simulink model "Parallel_n64"  (R2012b)
settings: Solver=VariableStepDiscrete  StartTime=0.0  StopTime=TotalIterations  RelTol=1e-3
values from neighbouring files (symbols this model uses):
  bp = 12    [ConfigValidate.m]
  bpSNMemory = bp    (= 12)    [ConfigValidate.m]
  IterationsOrdering = 4000    [ConfigValidate.m]
  MaxCoordDistance = (abs(max(wx) - min(wx))+abs(max(wy) - min(wy)))^2    [ConfigValidate.m]
  N_limit = 0.01    [ConfigValidate.m]
  nBits = 9    [ConfigValidate.m]
  nBitsNSmemories = (ceil(log2(TotalIterations)))    [ConfigValidate.m]
  S_limit = 1    [ConfigValidate.m]
  SourceNodes = 2000    [ConfigValidate.m]
  ts = 1    [ConfigValidate.m]
  w1 = rand(1,Neurons)    [ConfigValidate.m]
  w2 = rand(1,Neurons)    [ConfigValidate.m]
  wx = zeros(1,Neurons)    [ConfigValidate.m]
  wy = zeros(1,Neurons)    [ConfigValidate.m]
  x1 = rand(SourceNodes,1)    [ConfigValidate.m]
  x2 = rand(SourceNodes,1)    [ConfigValidate.m]
libraries: xbsIndex_r4 x6367, dspsrcs4 x2, dspstat3 x2
(part 2 of 28)

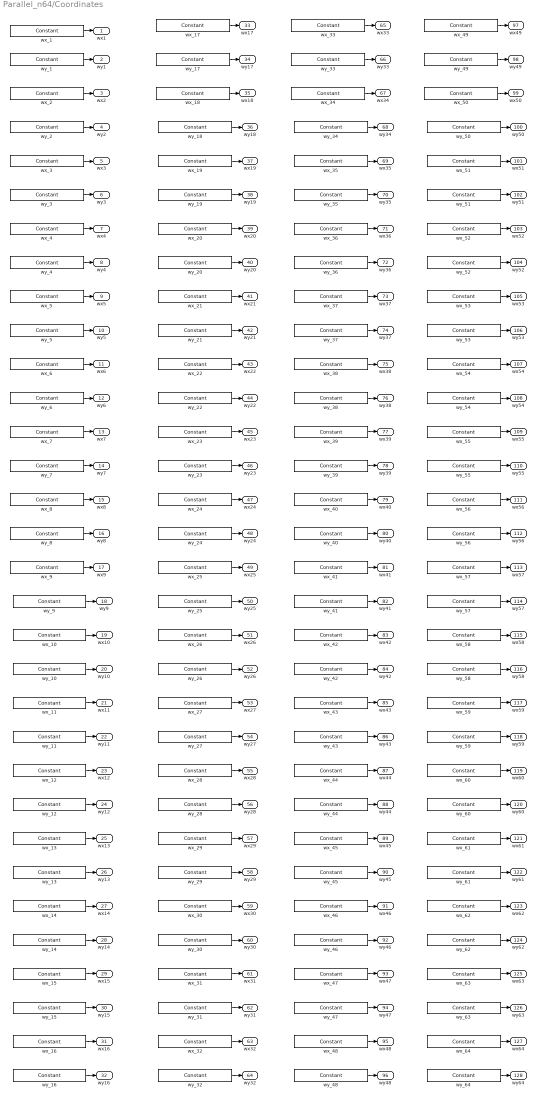
== system Parallel_n64/Coordinates ==
  wx_1 : xbsIndex_r4/Constant  const=wx(1)  gui_display_data_type=Fixed-point  arith_type=Unsigned  n_bits=nbCoord  bin_pt=bpCoord  preci_type=Single  exp_width=8  frac_width=24  explicit_period=on  period=ts  equ=P=C  opselect=C  inp2=PCIN>>17  opr=+  inp1=P  carry=CIN  dbl_ovrd=off  block_type=constant
  wx_{10,26,42,58} (4 alike) : xbsIndex_r4/Constant  const=wx(10)  gui_display_data_type=Fixed-point  arith_type=Unsigned  n_bits=nbCoord  bin_pt=bpCoord  preci_type=Single  exp_width=8  frac_width=24  explicit_period=on  period=ts  equ=P=C  opselect=C  inp2=PCIN>>17  opr=+  inp1=P  carry=CIN  dbl_ovrd=off  block_type=constant
  wx_{11,27,43,59} (4 alike) : xbsIndex_r4/Constant  const=wx(11)  gui_display_data_type=Fixed-point  arith_type=Unsigned  n_bits=nbCoord  bin_pt=bpCoord  preci_type=Single  exp_width=8  frac_width=24  explicit_period=on  period=ts  equ=P=C  opselect=C  inp2=PCIN>>17  opr=+  inp1=P  carry=CIN  dbl_ovrd=off  block_type=constant
  wx_{12,28,44,60} (4 alike) : xbsIndex_r4/Constant  const=wx(12)  gui_display_data_type=Fixed-point  arith_type=Unsigned  n_bits=nbCoord  bin_pt=bpCoord  preci_type=Single  exp_width=8  frac_width=24  explicit_period=on  period=ts  equ=P=C  opselect=C  inp2=PCIN>>17  opr=+  inp1=P  carry=CIN  dbl_ovrd=off  block_type=constant
  wx_{13,29,45,61} (4 alike) : xbsIndex_r4/Constant  const=wx(13)  gui_display_data_type=Fixed-point  arith_type=Unsigned  n_bits=nbCoord  bin_pt=bpCoord  preci_type=Single  exp_width=8  frac_width=24  explicit_period=on  period=ts  equ=P=C  opselect=C  inp2=PCIN>>17  opr=+  inp1=P  carry=CIN  dbl_ovrd=off  block_type=constant
  wx_{14,30,46,62} (4 alike) : xbsIndex_r4/Constant  const=wx(14)  gui_display_data_type=Fixed-point  arith_type=Unsigned  n_bits=nbCoord  bin_pt=bpCoord  preci_type=Single  exp_width=8  frac_width=24  explicit_period=on  period=ts  equ=P=C  opselect=C  inp2=PCIN>>17  opr=+  inp1=P  carry=CIN  dbl_ovrd=off  block_type=constant
  wx_{15,31,47,63} (4 alike) : xbsIndex_r4/Constant  const=wx(15)  gui_display_data_type=Fixed-point  arith_type=Unsigned  n_bits=nbCoord  bin_pt=bpCoord  preci_type=Single  exp_width=8  frac_width=24  explicit_period=on  period=ts  equ=P=C  opselect=C  inp2=PCIN>>17  opr=+  inp1=P  carry=CIN  dbl_ovrd=off  block_type=constant
  wx_{16,32,48,64} (4 alike) : xbsIndex_r4/Constant  const=wx(16)  gui_display_data_type=Fixed-point  arith_type=Unsigned  n_bits=nbCoord  bin_pt=bpCoord  preci_type=Single  exp_width=8  frac_width=24  explicit_period=on  period=ts  equ=P=C  opselect=C  inp2=PCIN>>17  opr=+  inp1=P  carry=CIN  dbl_ovrd=off  block_type=constant
  wx_17 : xbsIndex_r4/Constant  const=wx(17)  gui_display_data_type=Fixed-point  arith_type=Unsigned  n_bits=nbCoord  bin_pt=bpCoord  preci_type=Single  exp_width=8  frac_width=24  explicit_period=on  period=ts  equ=P=C  opselect=C  inp2=PCIN>>17  opr=+  inp1=P  carry=CIN  dbl_ovrd=off  block_type=constant
  wx_18 : xbsIndex_r4/Constant  const=wx(18)  gui_display_data_type=Fixed-point  arith_type=Unsigned  n_bits=nbCoord  bin_pt=bpCoord  preci_type=Single  exp_width=8  frac_width=24  explicit_period=on  period=ts  equ=P=C  opselect=C  inp2=PCIN>>17  opr=+  inp1=P  carry=CIN  dbl_ovrd=off  block_type=constant
  wx_19 : xbsIndex_r4/Constant  const=wx(19)  gui_display_data_type=Fixed-point  arith_type=Unsigned  n_bits=nbCoord  bin_pt=bpCoord  preci_type=Single  exp_width=8  frac_width=24  explicit_period=on  period=ts  equ=P=C  opselect=C  inp2=PCIN>>17  opr=+  inp1=P  carry=CIN  dbl_ovrd=off  block_type=constant
  wx_2 : xbsIndex_r4/Constant  const=wx(2)  gui_display_data_type=Fixed-point  arith_type=Unsigned  n_bits=nbCoord  bin_pt=bpCoord  preci_type=Single  exp_width=8  frac_width=24  explicit_period=on  period=ts  equ=P=C  opselect=C  inp2=PCIN>>17  opr=+  inp1=P  carry=CIN  dbl_ovrd=off  block_type=constant
  wx_20 : xbsIndex_r4/Constant  const=wx(20)  gui_display_data_type=Fixed-point  arith_type=Unsigned  n_bits=nbCoord  bin_pt=bpCoord  preci_type=Single  exp_width=8  frac_width=24  explicit_period=on  period=ts  equ=P=C  opselect=C  inp2=PCIN>>17  opr=+  inp1=P  carry=CIN  dbl_ovrd=off  block_type=constant
  wx_21 : xbsIndex_r4/Constant  const=wx(21)  gui_display_data_type=Fixed-point  arith_type=Unsigned  n_bits=nbCoord  bin_pt=bpCoord  preci_type=Single  exp_width=8  frac_width=24  explicit_period=on  period=ts  equ=P=C  opselect=C  inp2=PCIN>>17  opr=+  inp1=P  carry=CIN  dbl_ovrd=off  block_type=constant
  wx_22 : xbsIndex_r4/Constant  const=wx(22)  gui_display_data_type=Fixed-point  arith_type=Unsigned  n_bits=nbCoord  bin_pt=bpCoord  preci_type=Single  exp_width=8  frac_width=24  explicit_period=on  period=ts  equ=P=C  opselect=C  inp2=PCIN>>17  opr=+  inp1=P  carry=CIN  dbl_ovrd=off  block_type=constant
  wx_23 : xbsIndex_r4/Constant  const=wx(23)  gui_display_data_type=Fixed-point  arith_type=Unsigned  n_bits=nbCoord  bin_pt=bpCoord  preci_type=Single  exp_width=8  frac_width=24  explicit_period=on  period=ts  equ=P=C  opselect=C  inp2=PCIN>>17  opr=+  inp1=P  carry=CIN  dbl_ovrd=off  block_type=constant
  wx_24 : xbsIndex_r4/Constant  const=wx(24)  gui_display_data_type=Fixed-point  arith_type=Unsigned  n_bits=nbCoord  bin_pt=bpCoord  preci_type=Single  exp_width=8  frac_width=24  explicit_period=on  period=ts  equ=P=C  opselect=C  inp2=PCIN>>17  opr=+  inp1=P  carry=CIN  dbl_ovrd=off  block_type=constant
  wx_25 : xbsIndex_r4/Constant  const=wx(25)  gui_display_data_type=Fixed-point  arith_type=Unsigned  n_bits=nbCoord  bin_pt=bpCoord  preci_type=Single  exp_width=8  frac_width=24  explicit_period=on  period=ts  equ=P=C  opselect=C  inp2=PCIN>>17  opr=+  inp1=P  carry=CIN  dbl_ovrd=off  block_type=constant
  wx_3 : xbsIndex_r4/Constant  const=wx(3)  gui_display_data_type=Fixed-point  arith_type=Unsigned  n_bits=nbCoord  bin_pt=bpCoord  preci_type=Single  exp_width=8  frac_width=24  explicit_period=on  period=ts  equ=P=C  opselect=C  inp2=PCIN>>17  opr=+  inp1=P  carry=CIN  dbl_ovrd=off  block_type=constant
  wx_33 : xbsIndex_r4/Constant  const=wx(17)  gui_display_data_type=Fixed-point  arith_type=Unsigned  n_bits=nbCoord  bin_pt=bpCoord  preci_type=Single  exp_width=8  frac_width=24  explicit_period=on  period=ts  equ=P=C  opselect=C  inp2=PCIN>>17  opr=+  inp1=P  carry=CIN  dbl_ovrd=off  block_type=constant
  wx_34 : xbsIndex_r4/Constant  const=wx(18)  gui_display_data_type=Fixed-point  arith_type=Unsigned  n_bits=nbCoord  bin_pt=bpCoord  preci_type=Single  exp_width=8  frac_width=24  explicit_period=on  period=ts  equ=P=C  opselect=C  inp2=PCIN>>17  opr=+  inp1=P  carry=CIN  dbl_ovrd=off  block_type=constant
  wx_35 : xbsIndex_r4/Constant  const=wx(19)  gui_display_data_type=Fixed-point  arith_type=Unsigned  n_bits=nbCoord  bin_pt=bpCoord  preci_type=Single  exp_width=8  frac_width=24  explicit_period=on  period=ts  equ=P=C  opselect=C  inp2=PCIN>>17  opr=+  inp1=P  carry=CIN  dbl_ovrd=off  block_type=constant
  wx_36 : xbsIndex_r4/Constant  const=wx(20)  gui_display_data_type=Fixed-point  arith_type=Unsigned  n_bits=nbCoord  bin_pt=bpCoord  preci_type=Single  exp_width=8  frac_width=24  explicit_period=on  period=ts  equ=P=C  opselect=C  inp2=PCIN>>17  opr=+  inp1=P  carry=CIN  dbl_ovrd=off  block_type=constant
  wx_37 : xbsIndex_r4/Constant  const=wx(21)  gui_display_data_type=Fixed-point  arith_type=Unsigned  n_bits=nbCoord  bin_pt=bpCoord  preci_type=Single  exp_width=8  frac_width=24  explicit_period=on  period=ts  equ=P=C  opselect=C  inp2=PCIN>>17  opr=+  inp1=P  carry=CIN  dbl_ovrd=off  block_type=constant
  wx_38 : xbsIndex_r4/Constant  const=wx(22)  gui_display_data_type=Fixed-point  arith_type=Unsigned  n_bits=nbCoord  bin_pt=bpCoord  preci_type=Single  exp_width=8  frac_width=24  explicit_period=on  period=ts  equ=P=C  opselect=C  inp2=PCIN>>17  opr=+  inp1=P  carry=CIN  dbl_ovrd=off  block_type=constant
  wx_39 : xbsIndex_r4/Constant  const=wx(23)  gui_display_data_type=Fixed-point  arith_type=Unsigned  n_bits=nbCoord  bin_pt=bpCoord  preci_type=Single  exp_width=8  frac_width=24  explicit_period=on  period=ts  equ=P=C  opselect=C  inp2=PCIN>>17  opr=+  inp1=P  carry=CIN  dbl_ovrd=off  block_type=constant
  wx_4 : xbsIndex_r4/Constant  const=wx(4)  gui_display_data_type=Fixed-point  arith_type=Unsigned  n_bits=nbCoord  bin_pt=bpCoord  preci_type=Single  exp_width=8  frac_width=24  explicit_period=on  period=ts  equ=P=C  opselect=C  inp2=PCIN>>17  opr=+  inp1=P  carry=CIN  dbl_ovrd=off  block_type=constant
  wx_40 : xbsIndex_r4/Constant  const=wx(24)  gui_display_data_type=Fixed-point  arith_type=Unsigned  n_bits=nbCoord  bin_pt=bpCoord  preci_type=Single  exp_width=8  frac_width=24  explicit_period=on  period=ts  equ=P=C  opselect=C  inp2=PCIN>>17  opr=+  inp1=P  carry=CIN  dbl_ovrd=off  block_type=constant
  wx_41 : xbsIndex_r4/Constant  const=wx(25)  gui_display_data_type=Fixed-point  arith_type=Unsigned  n_bits=nbCoord  bin_pt=bpCoord  preci_type=Single  exp_width=8  frac_width=24  explicit_period=on  period=ts  equ=P=C  opselect=C  inp2=PCIN>>17  opr=+  inp1=P  carry=CIN  dbl_ovrd=off  block_type=constant
  wx_49 : xbsIndex_r4/Constant  const=wx(17)  gui_display_data_type=Fixed-point  arith_type=Unsigned  n_bits=nbCoord  bin_pt=bpCoord  preci_type=Single  exp_width=8  frac_width=24  explicit_period=on  period=ts  equ=P=C  opselect=C  inp2=PCIN>>17  opr=+  inp1=P  carry=CIN  dbl_ovrd=off  block_type=constant
  wx_5 : xbsIndex_r4/Constant  const=wx(5)  gui_display_data_type=Fixed-point  arith_type=Unsigned  n_bits=nbCoord  bin_pt=bpCoord  preci_type=Single  exp_width=8  frac_width=24  explicit_period=on  period=ts  equ=P=C  opselect=C  inp2=PCIN>>17  opr=+  inp1=P  carry=CIN  dbl_ovrd=off  block_type=constant
  wx_50 : xbsIndex_r4/Constant  const=wx(18)  gui_display_data_type=Fixed-point  arith_type=Unsigned  n_bits=nbCoord  bin_pt=bpCoord  preci_type=Single  exp_width=8  frac_width=24  explicit_period=on  period=ts  equ=P=C  opselect=C  inp2=PCIN>>17  opr=+  inp1=P  carry=CIN  dbl_ovrd=off  block_type=constant
  wx_51 : xbsIndex_r4/Constant  const=wx(19)  gui_display_data_type=Fixed-point  arith_type=Unsigned  n_bits=nbCoord  bin_pt=bpCoord  preci_type=Single  exp_width=8  frac_width=24  explicit_period=on  period=ts  equ=P=C  opselect=C  inp2=PCIN>>17  opr=+  inp1=P  carry=CIN  dbl_ovrd=off  block_type=constant
  wx_52 : xbsIndex_r4/Constant  const=wx(20)  gui_display_data_type=Fixed-point  arith_type=Unsigned  n_bits=nbCoord  bin_pt=bpCoord  preci_type=Single  exp_width=8  frac_width=24  explicit_period=on  period=ts  equ=P=C  opselect=C  inp2=PCIN>>17  opr=+  inp1=P  carry=CIN  dbl_ovrd=off  block_type=constant
  wx_53 : xbsIndex_r4/Constant  const=wx(21)  gui_display_data_type=Fixed-point  arith_type=Unsigned  n_bits=nbCoord  bin_pt=bpCoord  preci_type=Single  exp_width=8  frac_width=24  explicit_period=on  period=ts  equ=P=C  opselect=C  inp2=PCIN>>17  opr=+  inp1=P  carry=CIN  dbl_ovrd=off  block_type=constant
  wx_54 : xbsIndex_r4/Constant  const=wx(22)  gui_display_data_type=Fixed-point  arith_type=Unsigned  n_bits=nbCoord  bin_pt=bpCoord  preci_type=Single  exp_width=8  frac_width=24  explicit_period=on  period=ts  equ=P=C  opselect=C  inp2=PCIN>>17  opr=+  inp1=P  carry=CIN  dbl_ovrd=off  block_type=constant
  wx_55 : xbsIndex_r4/Constant  const=wx(23)  gui_display_data_type=Fixed-point  arith_type=Unsigned  n_bits=nbCoord  bin_pt=bpCoord  preci_type=Single  exp_width=8  frac_width=24  explicit_period=on  period=ts  equ=P=C  opselect=C  inp2=PCIN>>17  opr=+  inp1=P  carry=CIN  dbl_ovrd=off  block_type=constant
  wx_56 : xbsIndex_r4/Constant  const=wx(24)  gui_display_data_type=Fixed-point  arith_type=Unsigned  n_bits=nbCoord  bin_pt=bpCoord  preci_type=Single  exp_width=8  frac_width=24  explicit_period=on  period=ts  equ=P=C  opselect=C  inp2=PCIN>>17  opr=+  inp1=P  carry=CIN  dbl_ovrd=off  block_type=constant
  wx_57 : xbsIndex_r4/Constant  const=wx(25)  gui_display_data_type=Fixed-point  arith_type=Unsigned  n_bits=nbCoord  bin_pt=bpCoord  preci_type=Single  exp_width=8  frac_width=24  explicit_period=on  period=ts  equ=P=C  opselect=C  inp2=PCIN>>17  opr=+  inp1=P  carry=CIN  dbl_ovrd=off  block_type=constant
  wx_6 : xbsIndex_r4/Constant  const=wx(6)  gui_display_data_type=Fixed-point  arith_type=Unsigned  n_bits=nbCoord  bin_pt=bpCoord  preci_type=Single  exp_width=8  frac_width=24  explicit_period=on  period=ts  equ=P=C  opselect=C  inp2=PCIN>>17  opr=+  inp1=P  carry=CIN  dbl_ovrd=off  block_type=constant
  wx_7 : xbsIndex_r4/Constant  const=wx(7)  gui_display_data_type=Fixed-point  arith_type=Unsigned  n_bits=nbCoord  bin_pt=bpCoord  preci_type=Single  exp_width=8  frac_width=24  explicit_period=on  period=ts  equ=P=C  opselect=C  inp2=PCIN>>17  opr=+  inp1=P  carry=CIN  dbl_ovrd=off  block_type=constant
  wx_8 : xbsIndex_r4/Constant  const=wx(8)  gui_display_data_type=Fixed-point  arith_type=Unsigned  n_bits=nbCoord  bin_pt=bpCoord  preci_type=Single  exp_width=8  frac_width=24  explicit_period=on  period=ts  equ=P=C  opselect=C  inp2=PCIN>>17  opr=+  inp1=P  carry=CIN  dbl_ovrd=off  block_type=constant
  wx_9 : xbsIndex_r4/Constant  const=wx(9)  gui_display_data_type=Fixed-point  arith_type=Unsigned  n_bits=nbCoord  bin_pt=bpCoord  preci_type=Single  exp_width=8  frac_width=24  explicit_period=on  period=ts  equ=P=C  opselect=C  inp2=PCIN>>17  opr=+  inp1=P  carry=CIN  dbl_ovrd=off  block_type=constant
  wy_1 : xbsIndex_r4/Constant  const=wy(1)  gui_display_data_type=Fixed-point  arith_type=Unsigned  n_bits=nbCoord  bin_pt=bpCoord  preci_type=Single  exp_width=8  frac_width=24  explicit_period=on  period=ts  equ=P=C  opselect=C  inp2=PCIN>>17  opr=+  inp1=P  carry=CIN  dbl_ovrd=off  block_type=constant
  wy_{10,26,42,58} (4 alike) : xbsIndex_r4/Constant  const=wy(10)  gui_display_data_type=Fixed-point  arith_type=Unsigned  n_bits=nbCoord  bin_pt=bpCoord  preci_type=Single  exp_width=8  frac_width=24  explicit_period=on  period=ts  equ=P=C  opselect=C  inp2=PCIN>>17  opr=+  inp1=P  carry=CIN  dbl_ovrd=off  block_type=constant
  wy_{11,27,43,59} (4 alike) : xbsIndex_r4/Constant  const=wy(11)  gui_display_data_type=Fixed-point  arith_type=Unsigned  n_bits=nbCoord  bin_pt=bpCoord  preci_type=Single  exp_width=8  frac_width=24  explicit_period=on  period=ts  equ=P=C  opselect=C  inp2=PCIN>>17  opr=+  inp1=P  carry=CIN  dbl_ovrd=off  block_type=constant
  wy_{12,28,44,60} (4 alike) : xbsIndex_r4/Constant  const=wy(12)  gui_display_data_type=Fixed-point  arith_type=Unsigned  n_bits=nbCoord  bin_pt=bpCoord  preci_type=Single  exp_width=8  frac_width=24  explicit_period=on  period=ts  equ=P=C  opselect=C  inp2=PCIN>>17  opr=+  inp1=P  carry=CIN  dbl_ovrd=off  block_type=constant
  wy_{13,29,45,61} (4 alike) : xbsIndex_r4/Constant  const=wy(13)  gui_display_data_type=Fixed-point  arith_type=Unsigned  n_bits=nbCoord  bin_pt=bpCoord  preci_type=Single  exp_width=8  frac_width=24  explicit_period=on  period=ts  equ=P=C  opselect=C  inp2=PCIN>>17  opr=+  inp1=P  carry=CIN  dbl_ovrd=off  block_type=constant
  wy_{14,30,46,62} (4 alike) : xbsIndex_r4/Constant  const=wy(14)  gui_display_data_type=Fixed-point  arith_type=Unsigned  n_bits=nbCoord  bin_pt=bpCoord  preci_type=Single  exp_width=8  frac_width=24  explicit_period=on  period=ts  equ=P=C  opselect=C  inp2=PCIN>>17  opr=+  inp1=P  carry=CIN  dbl_ovrd=off  block_type=constant
  wy_{15,31,47,63} (4 alike) : xbsIndex_r4/Constant  const=wy(15)  gui_display_data_type=Fixed-point  arith_type=Unsigned  n_bits=nbCoord  bin_pt=bpCoord  preci_type=Single  exp_width=8  frac_width=24  explicit_period=on  period=ts  equ=P=C  opselect=C  inp2=PCIN>>17  opr=+  inp1=P  carry=CIN  dbl_ovrd=off  block_type=constant
  wy_{16,32,48,64} (4 alike) : xbsIndex_r4/Constant  const=wy(16)  gui_display_data_type=Fixed-point  arith_type=Unsigned  n_bits=nbCoord  bin_pt=bpCoord  preci_type=Single  exp_width=8  frac_width=24  explicit_period=on  period=ts  equ=P=C  opselect=C  inp2=PCIN>>17  opr=+  inp1=P  carry=CIN  dbl_ovrd=off  block_type=constant
  wy_17 : xbsIndex_r4/Constant  const=wy(17)  gui_display_data_type=Fixed-point  arith_type=Unsigned  n_bits=nbCoord  bin_pt=bpCoord  preci_type=Single  exp_width=8  frac_width=24  explicit_period=on  period=ts  equ=P=C  opselect=C  inp2=PCIN>>17  opr=+  inp1=P  carry=CIN  dbl_ovrd=off  block_type=constant
  wy_18 : xbsIndex_r4/Constant  const=wy(18)  gui_display_data_type=Fixed-point  arith_type=Unsigned  n_bits=nbCoord  bin_pt=bpCoord  preci_type=Single  exp_width=8  frac_width=24  explicit_period=on  period=ts  equ=P=C  opselect=C  inp2=PCIN>>17  opr=+  inp1=P  carry=CIN  dbl_ovrd=off  block_type=constant
  wy_19 : xbsIndex_r4/Constant  const=wy(19)  gui_display_data_type=Fixed-point  arith_type=Unsigned  n_bits=nbCoord  bin_pt=bpCoord  preci_type=Single  exp_width=8  frac_width=24  explicit_period=on  period=ts  equ=P=C  opselect=C  inp2=PCIN>>17  opr=+  inp1=P  carry=CIN  dbl_ovrd=off  block_type=constant
  wy_2 : xbsIndex_r4/Constant  const=wy(2)  gui_display_data_type=Fixed-point  arith_type=Unsigned  n_bits=nbCoord  bin_pt=bpCoord  preci_type=Single  exp_width=8  frac_width=24  explicit_period=on  period=ts  equ=P=C  opselect=C  inp2=PCIN>>17  opr=+  inp1=P  carry=CIN  dbl_ovrd=off  block_type=constant
  wy_20 : xbsIndex_r4/Constant  const=wy(20)  gui_display_data_type=Fixed-point  arith_type=Unsigned  n_bits=nbCoord  bin_pt=bpCoord  preci_type=Single  exp_width=8  frac_width=24  explicit_period=on  period=ts  equ=P=C  opselect=C  inp2=PCIN>>17  opr=+  inp1=P  carry=CIN  dbl_ovrd=off  block_type=constant
  wy_21 : xbsIndex_r4/Constant  const=wy(21)  gui_display_data_type=Fixed-point  arith_type=Unsigned  n_bits=nbCoord  bin_pt=bpCoord  preci_type=Single  exp_width=8  frac_width=24  explicit_period=on  period=ts  equ=P=C  opselect=C  inp2=PCIN>>17  opr=+  inp1=P  carry=CIN  dbl_ovrd=off  block_type=constant
  wy_22 : xbsIndex_r4/Constant  const=wy(22)  gui_display_data_type=Fixed-point  arith_type=Unsigned  n_bits=nbCoord  bin_pt=bpCoord  preci_type=Single  exp_width=8  frac_width=24  explicit_period=on  period=ts  equ=P=C  opselect=C  inp2=PCIN>>17  opr=+  inp1=P  carry=CIN  dbl_ovrd=off  block_type=constant
  wy_23 : xbsIndex_r4/Constant  const=wy(23)  gui_display_data_type=Fixed-point  arith_type=Unsigned  n_bits=nbCoord  bin_pt=bpCoord  preci_type=Single  exp_width=8  frac_width=24  explicit_period=on  period=ts  equ=P=C  opselect=C  inp2=PCIN>>17  opr=+  inp1=P  carry=CIN  dbl_ovrd=off  block_type=constant
  wy_24 : xbsIndex_r4/Constant  const=wy(24)  gui_display_data_type=Fixed-point  arith_type=Unsigned  n_bits=nbCoord  bin_pt=bpCoord  preci_type=Single  exp_width=8  frac_width=24  explicit_period=on  period=ts  equ=P=C  opselect=C  inp2=PCIN>>17  opr=+  inp1=P  carry=CIN  dbl_ovrd=off  block_type=constant
  wy_25 : xbsIndex_r4/Constant  const=wy(25)  gui_display_data_type=Fixed-point  arith_type=Unsigned  n_bits=nbCoord  bin_pt=bpCoord  preci_type=Single  exp_width=8  frac_width=24  explicit_period=on  period=ts  equ=P=C  opselect=C  inp2=PCIN>>17  opr=+  inp1=P  carry=CIN  dbl_ovrd=off  block_type=constant
  wy_3 : xbsIndex_r4/Constant  const=wy(3)  gui_display_data_type=Fixed-point  arith_type=Unsigned  n_bits=nbCoord  bin_pt=bpCoord  preci_type=Single  exp_width=8  frac_width=24  explicit_period=on  period=ts  equ=P=C  opselect=C  inp2=PCIN>>17  opr=+  inp1=P  carry=CIN  dbl_ovrd=off  block_type=constant
  wy_33 : xbsIndex_r4/Constant  const=wy(17)  gui_display_data_type=Fixed-point  arith_type=Unsigned  n_bits=nbCoord  bin_pt=bpCoord  preci_type=Single  exp_width=8  frac_width=24  explicit_period=on  period=ts  equ=P=C  opselect=C  inp2=PCIN>>17  opr=+  inp1=P  carry=CIN  dbl_ovrd=off  block_type=constant
  wy_34 : xbsIndex_r4/Constant  const=wy(18)  gui_display_data_type=Fixed-point  arith_type=Unsigned  n_bits=nbCoord  bin_pt=bpCoord  preci_type=Single  exp_width=8  frac_width=24  explicit_period=on  period=ts  equ=P=C  opselect=C  inp2=PCIN>>17  opr=+  inp1=P  carry=CIN  dbl_ovrd=off  block_type=constant
  wy_35 : xbsIndex_r4/Constant  const=wy(19)  gui_display_data_type=Fixed-point  arith_type=Unsigned  n_bits=nbCoord  bin_pt=bpCoord  preci_type=Single  exp_width=8  frac_width=24  explicit_period=on  period=ts  equ=P=C  opselect=C  inp2=PCIN>>17  opr=+  inp1=P  carry=CIN  dbl_ovrd=off  block_type=constant
  wy_36 : xbsIndex_r4/Constant  const=wy(20)  gui_display_data_type=Fixed-point  arith_type=Unsigned  n_bits=nbCoord  bin_pt=bpCoord  preci_type=Single  exp_width=8  frac_width=24  explicit_period=on  period=ts  equ=P=C  opselect=C  inp2=PCIN>>17  opr=+  inp1=P  carry=CIN  dbl_ovrd=off  block_type=constant
  wy_37 : xbsIndex_r4/Constant  const=wy(21)  gui_display_data_type=Fixed-point  arith_type=Unsigned  n_bits=nbCoord  bin_pt=bpCoord  preci_type=Single  exp_width=8  frac_width=24  explicit_period=on  period=ts  equ=P=C  opselect=C  inp2=PCIN>>17  opr=+  inp1=P  carry=CIN  dbl_ovrd=off  block_type=constant
  wy_38 : xbsIndex_r4/Constant  const=wy(22)  gui_display_data_type=Fixed-point  arith_type=Unsigned  n_bits=nbCoord  bin_pt=bpCoord  preci_type=Single  exp_width=8  frac_width=24  explicit_period=on  period=ts  equ=P=C  opselect=C  inp2=PCIN>>17  opr=+  inp1=P  carry=CIN  dbl_ovrd=off  block_type=constant
  wy_39 : xbsIndex_r4/Constant  const=wy(23)  gui_display_data_type=Fixed-point  arith_type=Unsigned  n_bits=nbCoord  bin_pt=bpCoord  preci_type=Single  exp_width=8  frac_width=24  explicit_period=on  period=ts  equ=P=C  opselect=C  inp2=PCIN>>17  opr=+  inp1=P  carry=CIN  dbl_ovrd=off  block_type=constant
  wy_4 : xbsIndex_r4/Constant  const=wy(4)  gui_display_data_type=Fixed-point  arith_type=Unsigned  n_bits=nbCoord  bin_pt=bpCoord  preci_type=Single  exp_width=8  frac_width=24  explicit_period=on  period=ts  equ=P=C  opselect=C  inp2=PCIN>>17  opr=+  inp1=P  carry=CIN  dbl_ovrd=off  block_type=constant
  wy_40 : xbsIndex_r4/Constant  const=wy(24)  gui_display_data_type=Fixed-point  arith_type=Unsigned  n_bits=nbCoord  bin_pt=bpCoord  preci_type=Single  exp_width=8  frac_width=24  explicit_period=on  period=ts  equ=P=C  opselect=C  inp2=PCIN>>17  opr=+  inp1=P  carry=CIN  dbl_ovrd=off  block_type=constant
  wy_41 : xbsIndex_r4/Constant  const=wy(25)  gui_display_data_type=Fixed-point  arith_type=Unsigned  n_bits=nbCoord  bin_pt=bpCoord  preci_type=Single  exp_width=8  frac_width=24  explicit_period=on  period=ts  equ=P=C  opselect=C  inp2=PCIN>>17  opr=+  inp1=P  carry=CIN  dbl_ovrd=off  block_type=constant
  wy_49 : xbsIndex_r4/Constant  const=wy(17)  gui_display_data_type=Fixed-point  arith_type=Unsigned  n_bits=nbCoord  bin_pt=bpCoord  preci_type=Single  exp_width=8  frac_width=24  explicit_period=on  period=ts  equ=P=C  opselect=C  inp2=PCIN>>17  opr=+  inp1=P  carry=CIN  dbl_ovrd=off  block_type=constant
  wy_5 : xbsIndex_r4/Constant  const=wy(5)  gui_display_data_type=Fixed-point  arith_type=Unsigned  n_bits=nbCoord  bin_pt=bpCoord  preci_type=Single  exp_width=8  frac_width=24  explicit_period=on  period=ts  equ=P=C  opselect=C  inp2=PCIN>>17  opr=+  inp1=P  carry=CIN  dbl_ovrd=off  block_type=constant
  wy_50 : xbsIndex_r4/Constant  const=wy(18)  gui_display_data_type=Fixed-point  arith_type=Unsigned  n_bits=nbCoord  bin_pt=bpCoord  preci_type=Single  exp_width=8  frac_width=24  explicit_period=on  period=ts  equ=P=C  opselect=C  inp2=PCIN>>17  opr=+  inp1=P  carry=CIN  dbl_ovrd=off  block_type=constant
  wy_51 : xbsIndex_r4/Constant  const=wy(19)  gui_display_data_type=Fixed-point  arith_type=Unsigned  n_bits=nbCoord  bin_pt=bpCoord  preci_type=Single  exp_width=8  frac_width=24  explicit_period=on  period=ts  equ=P=C  opselect=C  inp2=PCIN>>17  opr=+  inp1=P  carry=CIN  dbl_ovrd=off  block_type=constant
  wy_52 : xbsIndex_r4/Constant  const=wy(20)  gui_display_data_type=Fixed-point  arith_type=Unsigned  n_bits=nbCoord  bin_pt=bpCoord  preci_type=Single  exp_width=8  frac_width=24  explicit_period=on  period=ts  equ=P=C  opselect=C  inp2=PCIN>>17  opr=+  inp1=P  carry=CIN  dbl_ovrd=off  block_type=constant
  wy_53 : xbsIndex_r4/Constant  const=wy(21)  gui_display_data_type=Fixed-point  arith_type=Unsigned  n_bits=nbCoord  bin_pt=bpCoord  preci_type=Single  exp_width=8  frac_width=24  explicit_period=on  period=ts  equ=P=C  opselect=C  inp2=PCIN>>17  opr=+  inp1=P  carry=CIN  dbl_ovrd=off  block_type=constant
  wy_54 : xbsIndex_r4/Constant  const=wy(22)  gui_display_data_type=Fixed-point  arith_type=Unsigned  n_bits=nbCoord  bin_pt=bpCoord  preci_type=Single  exp_width=8  frac_width=24  explicit_period=on  period=ts  equ=P=C  opselect=C  inp2=PCIN>>17  opr=+  inp1=P  carry=CIN  dbl_ovrd=off  block_type=constant
  wy_55 : xbsIndex_r4/Constant  const=wy(23)  gui_display_data_type=Fixed-point  arith_type=Unsigned  n_bits=nbCoord  bin_pt=bpCoord  preci_type=Single  exp_width=8  frac_width=24  explicit_period=on  period=ts  equ=P=C  opselect=C  inp2=PCIN>>17  opr=+  inp1=P  carry=CIN  dbl_ovrd=off  block_type=constant
  wy_56 : xbsIndex_r4/Constant  const=wy(24)  gui_display_data_type=Fixed-point  arith_type=Unsigned  n_bits=nbCoord  bin_pt=bpCoord  preci_type=Single  exp_width=8  frac_width=24  explicit_period=on  period=ts  equ=P=C  opselect=C  inp2=PCIN>>17  opr=+  inp1=P  carry=CIN  dbl_ovrd=off  block_type=constant
  wy_57 : xbsIndex_r4/Constant  const=wy(25)  gui_display_data_type=Fixed-point  arith_type=Unsigned  n_bits=nbCoord  bin_pt=bpCoord  preci_type=Single  exp_width=8  frac_width=24  explicit_period=on  period=ts  equ=P=C  opselect=C  inp2=PCIN>>17  opr=+  inp1=P  carry=CIN  dbl_ovrd=off  block_type=constant
  wy_6 : xbsIndex_r4/Constant  const=wy(6)  gui_display_data_type=Fixed-point  arith_type=Unsigned  n_bits=nbCoord  bin_pt=bpCoord  preci_type=Single  exp_width=8  frac_width=24  explicit_period=on  period=ts  equ=P=C  opselect=C  inp2=PCIN>>17  opr=+  inp1=P  carry=CIN  dbl_ovrd=off  block_type=constant
  wy_7 : xbsIndex_r4/Constant  const=wy(7)  gui_display_data_type=Fixed-point  arith_type=Unsigned  n_bits=nbCoord  bin_pt=bpCoord  preci_type=Single  exp_width=8  frac_width=24  explicit_period=on  period=ts  equ=P=C  opselect=C  inp2=PCIN>>17  opr=+  inp1=P  carry=CIN  dbl_ovrd=off  block_type=constant
  wy_8 : xbsIndex_r4/Constant  const=wy(8)  gui_display_data_type=Fixed-point  arith_type=Unsigned  n_bits=nbCoord  bin_pt=bpCoord  preci_type=Single  exp_width=8  frac_width=24  explicit_period=on  period=ts  equ=P=C  opselect=C  inp2=PCIN>>17  opr=+  inp1=P  carry=CIN  dbl_ovrd=off  block_type=constant
  wy_9 : xbsIndex_r4/Constant  const=wy(9)  gui_display_data_type=Fixed-point  arith_type=Unsigned  n_bits=nbCoord  bin_pt=bpCoord  preci_type=Single  exp_width=8  frac_width=24  explicit_period=on  period=ts  equ=P=C  opselect=C  inp2=PCIN>>17  opr=+  inp1=P  carry=CIN  dbl_ovrd=off  block_type=constant
  wx1 : Outport
  wy1 : Outport  Port=2
  wx2 : Outport  Port=3
  wy2 : Outport  Port=4
  wx3 : Outport  Port=5
  wy3 : Outport  Port=6
  wx4 : Outport  Port=7
  wy4 : Outport  Port=8
  wx5 : Outport  Port=9
  wy5 : Outport  Port=10
  wx6 : Outport  Port=11
  wy6 : Outport  Port=12
  wx7 : Outport  Port=13
  wy7 : Outport  Port=14
  wx8 : Outport  Port=15
  wy8 : Outport  Port=16
  wx9 : Outport  Port=17
  wy9 : Outport  Port=18
  wx10 : Outport  Port=19
  wy10 : Outport  Port=20
  wx11 : Outport  Port=21
  wy11 : Outport  Port=22
  wx12 : Outport  Port=23
  wy12 : Outport  Port=24
  wx13 : Outport  Port=25
  wy13 : Outport  Port=26
  wx14 : Outport  Port=27
  wy14 : Outport  Port=28
  wx15 : Outport  Port=29
  wy15 : Outport  Port=30
  wx16 : Outport  Port=31
  wy16 : Outport  Port=32
  wx17 : Outport  Port=33
  wy17 : Outport  Port=34
  wx18 : Outport  Port=35
  wy18 : Outport  Port=36
  wx19 : Outport  Port=37
  wy19 : Outport  Port=38
  wx20 : Outport  Port=39
  wy20 : Outport  Port=40
  wx21 : Outport  Port=41
  wy21 : Outport  Port=42
  wx22 : Outport  Port=43
  wy22 : Outport  Port=44
  wx23 : Outport  Port=45
  wy23 : Outport  Port=46
  wx24 : Outport  Port=47
  wy24 : Outport  Port=48
  wx25 : Outport  Port=49
  wy25 : Outport  Port=50
  wx26 : Outport  Port=51
  wy26 : Outport  Port=52
  wx27 : Outport  Port=53
  wy27 : Outport  Port=54
  wx28 : Outport  Port=55
  wy28 : Outport  Port=56
  wx29 : Outport  Port=57
  wy29 : Outport  Port=58
  wx30 : Outport  Port=59
  wy30 : Outport  Port=60
  wx31 : Outport  Port=61
  wy31 : Outport  Port=62
  wx32 : Outport  Port=63
  wy32 : Outport  Port=64
  wx33 : Outport  Port=65
  wy33 : Outport  Port=66
  wx34 : Outport  Port=67
  wy34 : Outport  Port=68
  wx35 : Outport  Port=69
  wy35 : Outport  Port=70
  wx36 : Outport  Port=71
  wy36 : Outport  Port=72
  wx37 : Outport  Port=73
  wy37 : Outport  Port=74
  wx38 : Outport  Port=75
  wy38 : Outport  Port=76
  wx39 : Outport  Port=77
  wy39 : Outport  Port=78
  wx40 : Outport  Port=79
  wy40 : Outport  Port=80
  wx41 : Outport  Port=81
  wy41 : Outport  Port=82
  wx42 : Outport  Port=83
  wy42 : Outport  Port=84
  wx43 : Outport  Port=85
  wy43 : Outport  Port=86
  wx44 : Outport  Port=87
  wy44 : Outport  Port=88
  wx45 : Outport  Port=89
  wy45 : Outport  Port=90
  wx46 : Outport  Port=91
  wy46 : Outport  Port=92
  wx47 : Outport  Port=93
  wy47 : Outport  Port=94
  wx48 : Outport  Port=95
  wy48 : Outport  Port=96
  wx49 : Outport  Port=97
  wy49 : Outport  Port=98
  wx50 : Outport  Port=99
  wy50 : Outport  Port=100
  wx51 : Outport  Port=101
  wy51 : Outport  Port=102
  wx52 : Outport  Port=103
  wy52 : Outport  Port=104
  wx53 : Outport  Port=105
  wy53 : Outport  Port=106
  wx54 : Outport  Port=107
  wy54 : Outport  Port=108
  wx55 : Outport  Port=109
  wy55 : Outport  Port=110
  wx56 : Outport  Port=111
  wy56 : Outport  Port=112
  wx57 : Outport  Port=113
  wy57 : Outport  Port=114
  wx58 : Outport  Port=115
  wy58 : Outport  Port=116
  wx59 : Outport  Port=117
  wy59 : Outport  Port=118
  wx60 : Outport  Port=119
  wy60 : Outport  Port=120
  wx61 : Outport  Port=121
  wy61 : Outport  Port=122
  wx62 : Outport  Port=123
  wy62 : Outport  Port=124
  wx63 : Outport  Port=125
  wy63 : Outport  Port=126
  wx64 : Outport  Port=127
  wy64 : Outport  Port=128
  wires:
  wy_2/1 -> wy2/1
  wy_16/1 -> wy16/1
  wx_9/1 -> wx9/1
  wy_3/1 -> wy3/1
  wx_3/1 -> wx3/1
  wy_5/1 -> wy5/1
  wx_2/1 -> wx2/1
  wx_12/1 -> wx12/1
  wy_6/1 -> wy6/1
  wx_11/1 -> wx11/1
  wy_11/1 -> wy11/1
  wy_14/1 -> wy14/1
  wy_8/1 -> wy8/1
  wy_7/1 -> wy7/1
  wx_8/1 -> wx8/1
  wx_5/1 -> wx5/1
  wx_4/1 -> wx4/1
  wx_7/1 -> wx7/1
  wx_15/1 -> wx15/1
  wy_1/1 -> wy1/1
  wy_4/1 -> wy4/1
  wx_16/1 -> wx16/1
  wx_6/1 -> wx6/1
  wy_13/1 -> wy13/1
  wx_14/1 -> wx14/1
  wy_15/1 -> wy15/1
  wx_10/1 -> wx10/1
  wy_10/1 -> wy10/1
  wx_13/1 -> wx13/1
  wy_9/1 -> wy9/1
  wy_12/1 -> wy12/1
  wy_25/1 -> wy25/1
  wx_18/1 -> wx18/1
  wx_21/1 -> wx21/1
  wx_20/1 -> wx20/1
  wy_20/1 -> wy20/1
  wy_23/1 -> wy23/1
  wy_17/1 -> wy17/1
  wx_17/1 -> wx17/1
  wx_24/1 -> wx24/1
  wx_25/1 -> wx25/1
  wy_22/1 -> wy22/1
  wx_23/1 -> wx23/1
  wy_24/1 -> wy24/1
  wx_19/1 -> wx19/1
  wy_19/1 -> wy19/1
  wx_22/1 -> wx22/1
  wy_18/1 -> wy18/1
  wy_21/1 -> wy21/1
  wx_1/1 -> wx1/1
  wy_32/1 -> wy32/1
  wx_28/1 -> wx28/1
  wx_27/1 -> wx27/1
  wy_27/1 -> wy27/1
  wy_30/1 -> wy30/1
  wx_31/1 -> wx31/1
  wx_32/1 -> wx32/1
  wy_29/1 -> wy29/1
  wx_30/1 -> wx30/1
  wy_31/1 -> wy31/1
  wx_26/1 -> wx26/1
  wy_26/1 -> wy26/1
  wx_29/1 -> wx29/1
  wy_28/1 -> wy28/1
  wy_41/1 -> wy41/1
  wx_34/1 -> wx34/1
  wx_37/1 -> wx37/1
  wx_36/1 -> wx36/1
  wy_36/1 -> wy36/1
  wy_39/1 -> wy39/1
  wy_33/1 -> wy33/1
  wx_33/1 -> wx33/1
  wx_40/1 -> wx40/1
  wx_41/1 -> wx41/1
  wy_38/1 -> wy38/1
  wx_39/1 -> wx39/1
  wy_40/1 -> wy40/1
  wx_35/1 -> wx35/1
  wy_35/1 -> wy35/1
  wx_38/1 -> wx38/1
  wy_34/1 -> wy34/1
  wy_37/1 -> wy37/1
  wy_48/1 -> wy48/1
  wx_44/1 -> wx44/1
  wx_43/1 -> wx43/1
  wy_43/1 -> wy43/1
  wy_46/1 -> wy46/1
  wx_47/1 -> wx47/1
  wx_48/1 -> wx48/1
  wy_45/1 -> wy45/1
  wx_46/1 -> wx46/1
  wy_47/1 -> wy47/1
  wx_42/1 -> wx42/1
  wy_42/1 -> wy42/1
  wx_45/1 -> wx45/1
  wy_44/1 -> wy44/1
  wy_57/1 -> wy57/1
  wx_50/1 -> wx50/1
  wx_53/1 -> wx53/1
  wx_52/1 -> wx52/1
  wy_52/1 -> wy52/1
  wy_55/1 -> wy55/1
  wy_49/1 -> wy49/1
  wx_49/1 -> wx49/1
  wx_56/1 -> wx56/1
  wx_57/1 -> wx57/1
  wy_54/1 -> wy54/1
  wx_55/1 -> wx55/1
  wy_56/1 -> wy56/1
  wx_51/1 -> wx51/1
  wy_51/1 -> wy51/1
  wx_54/1 -> wx54/1
  wy_50/1 -> wy50/1
  wy_53/1 -> wy53/1
  wy_64/1 -> wy64/1
  wx_60/1 -> wx60/1
  wx_59/1 -> wx59/1
  wy_59/1 -> wy59/1
  wy_62/1 -> wy62/1
  wx_63/1 -> wx63/1
  wx_64/1 -> wx64/1
  wy_61/1 -> wy61/1
  wx_62/1 -> wx62/1
  wy_63/1 -> wy63/1
  wx_58/1 -> wx58/1
  wy_58/1 -> wy58/1
  wx_61/1 -> wx61/1
  wy_60/1 -> wy60/1
